simulink model "RoutingTest"  (R2018b)
settings: Solver=VariableStepAuto  StartTime=0.0  StopTime=100  RelTol=1e-3
StartFcn:
  | coder.extrinsic('evalin');
  | coder.extrinsic('strcat');
  | 
  | productInstances = [];
  | productIDs = [];
  | 
  | evalin('base', 'productTypeIDSet = {''ProductW001'', ''ProductW002'',''ProductX001'', ''ProductY001'', ''ProductZ001'', ''ProductX002'', ''ProductY002'', ''ProductZ002''};' );
  | evalin('base', 'productTypeIDSet = string(productTypeIDSet);');
  | 
  | numProd = evalin('base', 'length(productTypeIDSet)');
  | evalin('base', 'serviceTime = [rand(5,5,numProd) < 1].*[1+0.3*randn(5,5,numProd)];');
  | 
  | evalin('base', strcat('RoutingController = Controller; RoutingController.Routing = SimpleRouting;'));
  | 
  | evalin('base', 'machine1 = Machine(1); RoutingController.createResourceListener(machine1);');
  | evalin('base', 'machine2 = Machine(2); RoutingController.createResourceListener(machine2);');
  | evalin('base', 'machine3 = Machine(3); RoutingController.createResourceListener(machine3);');
  | evalin('base', 'machine4 = Machine(4); RoutingController.createResourceListener(machine4);');
undefined symbols (not defined in the file or in its folder): m
settings Model: Creator=tas5  LastModifiedBy=tas5

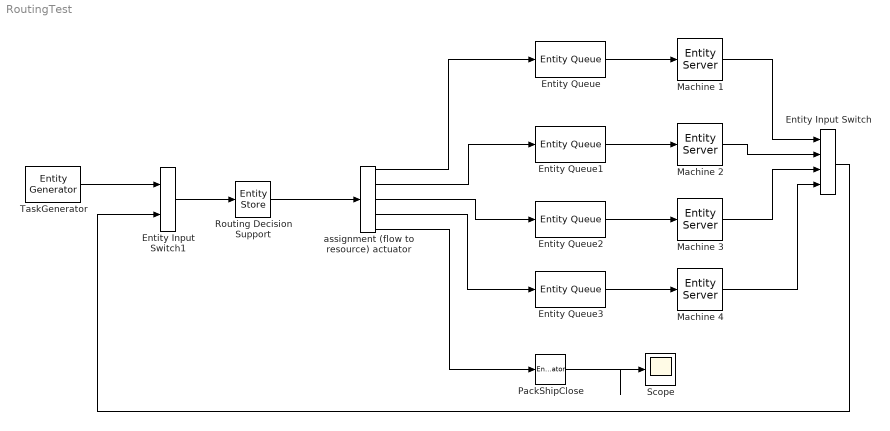
== system RoutingTest ==
  Entity Input Switch : EntityInputSwitch  InputPortMessageModes=m,m,m,m  OutputPortMessageModes=m  NumberInputPorts=4
      settings: InputPortMap=u1,u2,u3,u4
  Entity Input Switch1 : EntityInputSwitch  InputPortMessageModes=m,m  OutputPortMessageModes=m
  Entity Queue{,1..3} (4 alike) : EntityQueue  InputPortMessageModes=m  OutputPortMessageModes=m  QueueType=Priority  PrioritySource=enterTime
      settings: OutputPortMap=o5
  Machine 1 : EntityServer  InputPortMessageModes=m  OutputPortMessageModes=m  Capacity=1  ServiceTimeSource=Attribute  ServiceTimeAction=|  EntryAction=|  ServiceCompleteAction=|
      | coder.extrinsic('evalin');
      | 
      | dt = evalin('base', 'serviceTime(
      | coder.extrinsic('evalin')
      | coder.extrinsic('strcat');
      | coder.extrinsic('num2str');
      | 
      | 
      | %entity.ServiceTime = serviceTime(MachineType,ProcessType,ProductType);
      | entity.ServiceTime = evalin('base', strcat('serviceTime(', num2str(entity.nextNode), ...
      |     ', productInstances{[productIDs == ', num2str(entity.serialNumber), ']}.processPlan.currentProcessStep,', ...
      |     num2str(entity.productTypeID), ');'));
      | 
      | evalin('base', strcat('part = productInstances{[productIDs == ', num2str(entity.serialNumber), ']};', ...
      |     'part.currentProcessStep.actualStartTime = get_param(''RoutingTest'',''SimulationTime'');', ...
      |     'part.currentProcessStep.actualResource =', num2str(1),';'));
      | coder.extrinsic('evalin')
      | coder.extrinsic('strcat');
      | coder.extrinsic('num2str');
      | 
      | evalin('base', strcat('part = productInstances{[productIDs == ', num2str(entity.serialNumber), ']};', ...
      |     'part.currentProcessStep.actualCompleteTime = get_param(''RoutingTest'',''SimulationTime'');'));
      | 
      | coder.extrinsic('probInduceDefect');
      | coder.extrinsic('machineHealthIndex');
      | 
      | % Equipment health
      | persistent healthIndex;
      | persistent runTime;
      | persistent partCount;
      | if isempty(healthIndex)
      |         %Initial health level.
      |     healthIndex = 5;
      | end
      | if isempty(runTime)
      |     runTime = 0;
      | end
      | if isempty(partCount)
      |     partCount = 0;
      | end
      | 
      | runTime = runTime + entity.ServiceTime;
      | partCount = partCount + 1;
      | maxRunTime = 1500;
      | maxPartCount = 1000;
      | maxHealthIndex = 10;
      | healthIndex = machineHealthIndex(1, healthIndex,maxHealthIndex, runTime, maxRunTime, partCount, maxPartCount);
      | 
      | if healthIndex >= maxHealthIndex
      |     entity.condition = probInduceDefect(entity.condition, maxHealthIndex, entity.serialNumber);
      |     healthIndex = 2;
      | else
      |     entity.condition = probInduceDefect(entity.condition, healthIndex, entity.serialNumber);
      | end
      | 
      | % Write part condition to part
      | evalin('base', strcat('part = productInstances{[productIDs == ', num2str(entity.serialNumber), ']};', ...
      |     'part.actualOutputCondition = ', num2str(entity.condition),';'));
      | 
      | %Write machine condition to machine
      | evalin('base', strcat('machine1.machineHealth = ', num2str(healthIndex), ''));
  Machine 2 : EntityServer  InputPortMessageModes=m  OutputPortMessageModes=m  Capacity=1  ServiceTimeSource=Attribute  ServiceTimeAction=|  EntryAction=|  ServiceCompleteAction=|
      | coder.extrinsic('evalin');
      | 
      | dt = evalin('base', 'serviceTime(
      | coder.extrinsic('evalin')
      | coder.extrinsic('strcat');
      | coder.extrinsic('num2str');
      | 
      | %entity.ServiceTime = serviceTime(MachineType,ProcessType,ProductType);
      | entity.ServiceTime = evalin('base', strcat('serviceTime(', num2str(entity.nextNode), ...
      |     ', productInstances{[productIDs == ', num2str(entity.serialNumber), ']}.processPlan.currentProcessStep,', ...
      |     num2str(entity.productTypeID), ');'));
      | 
      | evalin('base', strcat('part = productInstances{[productIDs == ', num2str(entity.serialNumber), ']};', ...
      |     'part.currentProcessStep.actualStartTime = get_param(''RoutingTest'',''SimulationTime'');', ...
      |     'part.currentProcessStep.actualResource =', num2str(2),';'));
      | coder.extrinsic('evalin')
      | coder.extrinsic('strcat');
      | coder.extrinsic('num2str');
      | 
      | evalin('base', strcat('part = productInstances{[productIDs == ', num2str(entity.serialNumber), ']};', ...
      |     'part.currentProcessStep.actualCompleteTime = get_param(''RoutingTest'',''SimulationTime'');'));
      | 
      | coder.extrinsic('probInduceDefect');
      | coder.extrinsic('machineHealthIndex');
      | 
      | % Equipment health
      | persistent healthIndex;
      | persistent runTime;
      | persistent partCount;
      | if isempty(healthIndex)
      |         %Initial health level.
      |     healthIndex = 3;
      | end
      | if isempty(runTime)
      |     runTime = 0;
      | end
      | if isempty(partCount)
      |     partCount = 0;
      | end
      | 
      | runTime = runTime + entity.ServiceTime;
      | partCount = partCount + 1;
      | maxRunTime = 1000;
      | maxPartCount = 1000;
      | maxHealthIndex = 10;
      | healthIndex = machineHealthIndex(2 ,healthIndex,maxHealthIndex, runTime, maxRunTime, partCount, maxPartCount);
      | 
      | if healthIndex >= maxHealthIndex
      |     entity.condition = probInduceDefect(entity.condition, maxHealthIndex, entity.serialNumber);
      |     healthIndex = 2;
      | else
      |     entity.condition = probInduceDefect(entity.condition, healthIndex, entity.serialNumber);
      | end
      | 
      | % Write part condition to part
      | evalin('base', strcat('part = productInstances{[productIDs == ', num2str(entity.serialNumber), ']};', ...
      |     'part.actualOutputCondition = ', num2str(entity.condition),';'));
      | 
      | 
      | %Write machine condition to machine
      | evalin('base', strcat('machine2.machineHealth = ', num2str(healthIndex), ''));
  Machine 3 : EntityServer  InputPortMessageModes=m  OutputPortMessageModes=m  Capacity=1  ServiceTimeSource=Attribute  ServiceTimeAction=|  EntryAction=|  ServiceCompleteAction=|
      | coder.extrinsic('evalin');
      | 
      | dt = evalin('base', 'serviceTime(
      | coder.extrinsic('evalin')
      | coder.extrinsic('strcat');
      | coder.extrinsic('num2str');
      | 
      | %entity.ServiceTime = serviceTime(MachineType,ProcessType,ProductType);
      | entity.ServiceTime = evalin('base', strcat('serviceTime(', num2str(entity.nextNode), ...
      |     ', productInstances{[productIDs == ', num2str(entity.serialNumber), ']}.processPlan.currentProcessStep,', ...
      |     num2str(entity.productTypeID), ');'));
      | 
      | evalin('base', strcat('part = productInstances{[productIDs == ', num2str(entity.serialNumber), ']};', ...
      |     'part.currentProcessStep.actualStartTime = get_param(''RoutingTest'',''SimulationTime'');', ...
      |     'part.currentProcessStep.actualResource =', num2str(3),';'));
      | coder.extrinsic('evalin')
      | coder.extrinsic('strcat');
      | coder.extrinsic('num2str');
      | 
      | evalin('base', strcat('part = productInstances{[productIDs == ', num2str(entity.serialNumber), ']};', ...
      |     'part.currentProcessStep.actualCompleteTime = get_param(''RoutingTest'',''SimulationTime'');'));
      | 
      | coder.extrinsic('probInduceDefect');
      | coder.extrinsic('machineHealthIndex');
      | 
      | % Equipment health
      | persistent healthIndex;
      | persistent runTime;
      | persistent partCount;
      | if isempty(healthIndex)
      |         %Initial health level.
      |     healthIndex = 3;
      | end
      | if isempty(runTime)
      |     runTime = 0;
      | end
      | if isempty(partCount)
      |     partCount = 0;
      | end
      | 
      | runTime = runTime + entity.ServiceTime;
      | partCount = partCount + 1;
      | maxRunTime = 1500;
      | maxPartCount = 1000;
      | maxHealthIndex = 10;
      | healthIndex = machineHealthIndex(3 ,healthIndex,maxHealthIndex, runTime, maxRunTime, partCount, maxPartCount);
      | 
      | if healthIndex >= maxHealthIndex
      |     entity.condition = probInduceDefect(entity.condition, maxHealthIndex, entity.serialNumber);
      |     healthIndex = 2;
      | else
      |     entity.condition = probInduceDefect(entity.condition, healthIndex, entity.serialNumber);
      | end
      | 
      | % Write part condition to part
      | evalin('base', strcat('part = productInstances{[productIDs == ', num2str(entity.serialNumber), ']};', ...
      |     'part.actualOutputCondition = ', num2str(entity.condition),';'));
  Machine 4 : EntityServer  InputPortMessageModes=m  OutputPortMessageModes=m  Capacity=1  ServiceTimeSource=Attribute  ServiceTimeAction=|  EntryAction=|  ServiceCompleteAction=|
      | coder.extrinsic('evalin');
      | 
      | dt = evalin('base', 'serviceTime(
      | coder.extrinsic('evalin')
      | coder.extrinsic('strcat');
      | coder.extrinsic('num2str');
      | 
      | %entity.ServiceTime = serviceTime(MachineType,ProcessType,ProductType);
      | entity.ServiceTime = evalin('base', strcat('serviceTime(', num2str(entity.nextNode), ...
      |     ', productInstances{[productIDs == ', num2str(entity.serialNumber), ']}.processPlan.currentProcessStep,', ...
      |     num2str(entity.productTypeID), ');'));
      | 
      | evalin('base', strcat('part = productInstances{[productIDs == ', num2str(entity.serialNumber), ']};', ...
      |     'part.currentProcessStep.actualStartTime = get_param(''RoutingTest'',''SimulationTime'');', ...
      |     'part.currentProcessStep.actualResource =', num2str(4),';'));
      | coder.extrinsic('evalin')
      | coder.extrinsic('strcat');
      | coder.extrinsic('num2str');
      | 
      | evalin('base', strcat('part = productInstances{[productIDs == ', num2str(entity.serialNumber), ']};', ...
      |     'part.currentProcessStep.actualCompleteTime = get_param(''RoutingTest'',''SimulationTime'');'));
      | 
      | coder.extrinsic('probInduceDefect');
      | coder.extrinsic('machineHealthIndex');
      | 
      | % Equipment health
      | persistent healthIndex;
      | persistent runTime;
      | persistent partCount;
      | if isempty(healthIndex)
      |         %Initial health level.
      |     healthIndex = 2;
      | end
      | if isempty(runTime)
      |     runTime = 0;
      | end
      | if isempty(partCount)
      |     partCount = 0;
      | end
      | 
      | runTime = runTime + entity.ServiceTime;
      | partCount = partCount + 1;
      | maxRunTime = 1250;
      | maxPartCount = 1000;
      | maxHealthIndex = 10;
      | healthIndex = machineHealthIndex(4 ,healthIndex,maxHealthIndex, runTime, maxRunTime, partCount, maxPartCount);
      | 
      | if healthIndex >= maxHealthIndex
      |     entity.condition = probInduceDefect(entity.condition, maxHealthIndex, entity.serialNumber);
      |     healthIndex = 2;
      | else
      |     entity.condition = probInduceDefect(entity.condition, healthIndex, entity.serialNumber);
      | end
      | 
      | % Write part condition to part
      | evalin('base', strcat('part = productInstances{[productIDs == ', num2str(entity.serialNumber), ']};', ...
      |     'part.actualOutputCondition = ', num2str(entity.condition),';'));
  PackShipClose : EntityTerminator  InputPortMessageModes=m  EntryAction=|  NumberEntitiesArrived=on
      | coder.extrinsic('evalin')
      | coder.extrinsic('strcat')
      | coder.extrinsic('num2str')
      | 
      | simTime = evalin('base', 'get_param(''RoutingTest'',''SimulationTime'');');
      | evalin('base', strcat('part = productInstances{[productIDs == ', num2str(entity.serialNumber), ']};', ...
      |     'part.actualCompleteTime = ', num2str(simTime), ';', ...
      |     'part.processPlan.actualCompleteTime = ', num2str(simTime), ';', ...
      |     'part.currentProcessStep.actualCompleteTime = ', num2str(simTime), ';', ...
      |     'part.currentProcessStep.actualStartTime = ', num2str(simTime), ';', ...
      |     'part.currentProcessStep.typeID = ''PackShipClose'' ;', ...
      |     'part.actualOutputCondition = ', num2str(entity.condition,5), ';'));
      |     
      |     evalin('base', strcat('part = productInstances{[productIDs == ', num2str(entity.serialNumber), ']};', ...
      |     'part.currentProcessStep.actualCompleteTime = get_param(''RoutingTest'',''SimulationTime'');'));
      settings: OutputPortMap=o0
  Routing Decision Support : EntityStore  InitFcn=|  InputPortMessageModes=m  OutputPortMessageModes=m  Capacity=1  EntryAction=|
      | coder.extrinsic('evalin')
      | 
      | evalin('base', 'RoutingController = Controller;')
      | evalin('base','RoutingController.Routing = SimpleRouting;');
      | coder.extrinsic('evalin')
      | coder.extrinsic('strcat')
      | coder.extrinsic('num2str')
      | 
      | 
      | entity.nextNode = evalin('base', strcat('RoutingController.Routing.Routing(productInstances{[productIDs == ', num2str(entity.serialNumber), ']})'));
      settings: OutputPortMap=o4
  Scope : Scope
  TaskGenerator : EntityGenerator  OutputPortMessageModes=m  Period=2.5  GenerateAction=|  ExitAction=|  AttributeName=productTypeID|serialNumber|nextNode|ServiceTime|condition|enterTime  AttributeInitialValue=1|1|5|1|1|1  EntityType=Structured  EntityTypeName=Task
      GenerateAction=|
      | coder.extrinsic('randi');
      | coder.extrinsic('evalin');
      | persistent idx;
      | persistent rngInit;
      | if isempty(idx)
      |     idx = 1;
      | end
      | if isempty(rngInit)
      |     seed = 12345;
      |     rng(seed);
      |     rngInit = true;
      | end
      | 
      | % Pattern: Arbitrary discrete distribution
      | % V: Value vector
      | % P: Probability vector
      | entity.productTypeID = randi(8);
      | 
      | entity.serialNumber = idx;
      | idx = idx + 1;
      | 
      | entity.enterTime = evalin('base', 'get_param(''RoutingTest'',''SimulationTime'');');
      ExitAction=|
      | coder.extrinsic('evalin')
      | coder.extrinsic('strcat')
      | coder.extrinsic('num2str')
      | 
      | %productTypeIDSet = evalin('base', 'productTypeIDSet');
      | productTypeIDSet = {'ProductW001', 'ProductW002','ProductX001', 'ProductY001', 'ProductZ001', 'ProductX002', 'ProductY002', 'ProductZ002'};
      | 
      | productTypeID = productTypeIDSet{entity.productTypeID};
      | evalin('base', strcat('productInstances{end+1} = ', productTypeID, '(', num2str(entity.serialNumber), ');'));
      | evalin('base', strcat('productIDs(end+1) = ', num2str(entity.serialNumber), ';'));
      | 
      | evalin('base', strcat('part = productInstances{[productIDs == ', num2str(entity.serialNumber), ']};', ...
      |     'RoutingController.createProductListener(part);', ...    
      |     'part.processPlan.actualStartTime = get_param(''RoutingTest'',''SimulationTime'');'));
  assignment (flow to resource) actuator : EntityOutputSwitch  InputPortMessageModes=m  OutputPortMessageModes=m,m,m,m,m  NumberOutputPorts=5  SwitchingCriterion=From attribute  SwitchAttributeName=nextNode
      settings: OutputPortMap=o0,o1,o2,o3,o4
  wires:
  Entity Queue/1 -> Machine 1/1
  Entity Queue1/1 -> Machine 2/1
  Entity Queue2/1 -> Machine 3/1
  Entity Queue3/1 -> Machine 4/1
  assignment (flow to resource) actuator/5 -> PackShipClose/1
  assignment (flow to resource) actuator/4 -> Entity Queue3/1
  assignment (flow to resource) actuator/3 -> Entity Queue2/1
  assignment (flow to resource) actuator/2 -> Entity Queue1/1
  assignment (flow to resource) actuator/1 -> Entity Queue/1
  Machine 1/1 -> Entity Input Switch/1
  Machine 2/1 -> Entity Input Switch/2
  Machine 3/1 -> Entity Input Switch/3
  Machine 4/1 -> Entity Input Switch/4
  TaskGenerator/1 -> Entity Input Switch1/1
  Entity Input Switch/1 -> Entity Input Switch1/2
  Entity Input Switch1/1 -> Routing Decision Support/1
  Routing Decision Support/1 -> assignment (flow to resource) actuator/1
  PackShipClose/1 -> Scope/1
